simulink model "three_chessclock_v2"  (R2018b)
settings: Solver=VariableStepAuto  StartTime=0.0  StopTime=inf  RelTol=1e-3
libraries: three_chessclock_library x2
settings Model: EnablePacing=on  PacingRate=10  Creator=svdh  LastModifiedBy=svdh

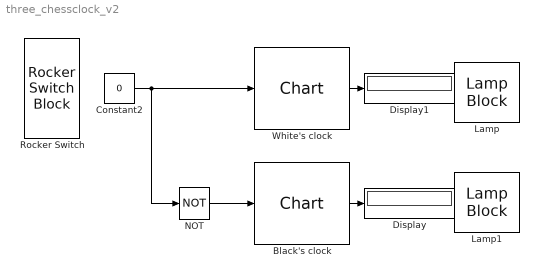
== system three_chessclock_v2 ==
  Black's clock : three_chessclock_library/Chart  SystemSampleTime=-1
  Constant2 : Constant  Value=0
  Display : Display
  Display1 : Display
  Lamp : LampBlock  WebBlockId=3
  Lamp1 : LampBlock  WebBlockId=4
  NOT : Logic  Operator=NOT  IconShape=distinctive  AllPortsSameDT=off  OutDataTypeStr=boolean
  Rocker Switch : RockerSwitchBlock  WebBlockId=6
      settings: Values={{'Black''s turn', 'White''s turn'}, [0 1]}
  White's clock : three_chessclock_library/Chart  SystemSampleTime=-1
  wires:
  Constant2/1 -> White's clock/1, NOT/1
  NOT/1 -> Black's clock/1
  Black's clock/1 -> Display/1
  White's clock/1 -> Display1/1
